simulink model "NREL_5MW_Controller_x86"  (R2019b)
settings: Solver=ode4  StartTime=0.0  StopTime=TMax  FixedStep=DT  MaxStep=DT  RelTol=1e-3  EnableMultiTasking=on
InitFcn:
  | Lambda_ref = 5;
values from neighbouring files (symbols this model uses):
  OutList =     [OutList.mat]
undefined symbols (not defined in the file or in its folder): pitch_cmd, rotor_cmd, strmatch
CloseFcn:
  | olist = OutList;
settings Model: Creator=bjonkman  LastModifiedBy=arthu
settings DataIOCC: SaveFormat=Array  SignalLoggingSaveFormat=ModelDataLogs  SaveOutput=off  SaveTime=off  ReturnWorkspaceOutputs=off  SignalLoggingName=sigsOut
settings OptimizationCC: ExpressionDepthLimit=2147483647  LifeSpan=inf
settings DebuggingCC: SaveWithParameterizedLinksMsg=none  UnderspecifiedInitializationDetection=Classic  MergeDetectMultiDrivingBlocksExec=none  SignalResolutionControl=TryResolveAllWithWarning  MultiTaskDSMMsg=warning  MultiTaskCondExecSysMsg=none  FcnCallInpInsideContextMsg=warning  StateNameClashWarn=warning  SFUnexpectedBacktrackingDiag=warning  SFNoUnconditionalDefaultTransitionDiag=warning  SFExecutionAtInitializationDiag=none  ArithmeticOperatorsInVariantConditions=warning
settings HardwareCC: ProdBitPerPointer=32  ProdBitPerSizeT=32  ProdBitPerPtrDiffT=32  ProdLargestAtomicFloat=None  ProdIntDivRoundTo=Undefined  ProdEndianess=Unspecified  ProdWordSize=32  ProdHWDeviceType=32-bit Generic  TargetUnknown=on
settings ModelReferenceCC: PropagateSignalLabelsOutOfModel=off
settings SFSimCC: SimUseLocalCustomCode=off  CustomCodeUndefinedFunction=UseInterfaceOnly
settings RTWCC: RTWUseLocalCustomCode=off
settings CodeAppCC: StateflowObjectComments=on
settings GRTTargetCC: TargetLangStandard=C89/C90 (ANSI)  ModelReferenceCompliant=off  ParMdlRefBuildCompliant=off  CompOptLevelCompliant=off  ConcurrentExecutionCompliant=off  CombineOutputUpdateFcns=off  MatFileLogging=off  GRTInterface=on
settings ConfigComp: CovMetricSettings=dw  CovHtmlReporting=on  CovSaveCumulativeToWorkspaceVar=on  CovSaveSingleToWorkspaceVar=on  CovExternalEMLEnable=off

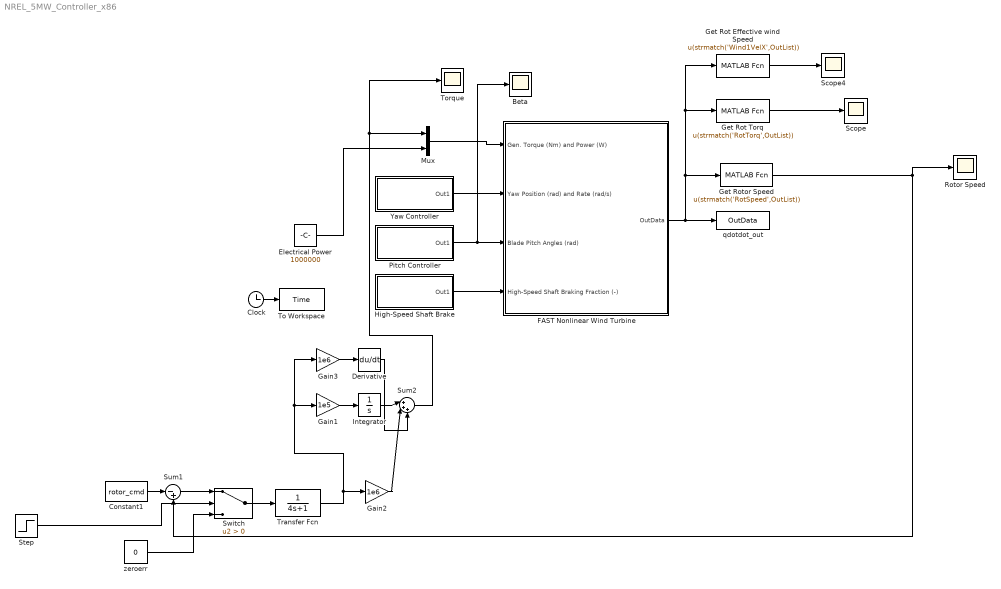
== system NREL_5MW_Controller_x86 ==
  Beta : Scope
  Clock : Clock
  Constant1 : Constant  Value=rotor_cmd
  Derivative : Derivative  CoefficientInTFapproximation=100
  Electrical Power : Constant  Value=1000000
  FAST Nonlinear Wind Turbine : Subsystem  mask(FAST Nonlinear Wind Turbine){}
      mask help: This block contains the FAST S-Function.
      mask init:
      | clear FAST_SFunc
  Gain1 : Gain  Gain=1e5
  Gain2 : Gain  Gain=1e6
  Gain3 : Gain  Gain=1e6
  Get Rot Effective wind Speed : MATLABFcn  MATLABFcn=u(strmatch('Wind1VelX',OutList))
  Get Rot Torq : MATLABFcn  MATLABFcn=u(strmatch('RotTorq',OutList))
  Get Rotor Speed : MATLABFcn  MATLABFcn=u(strmatch('RotSpeed',OutList))
  High-Speed Shaft Brake : Subsystem
  Integrator : Integrator
  Mux : Mux  Inputs=2
  Pitch Controller : Subsystem
  Rotor Speed : Scope
  Scope : Scope
  Scope4 : Scope
  Step : Step  Time=10  Before=-1  SampleTime=0
  Sum1 : Sum  Inputs=|-+
  Sum2 : Sum  Inputs=|+++
  Switch : Switch  Criteria=u2 > Threshold
  To Workspace : ToWorkspace  VariableName=Time  SampleTime=-1
  Torque : Scope
  Transfer Fcn : TransferFcn  Denominator=[4 1]
  Yaw Controller : Subsystem
  qdotdot_out : ToWorkspace  VariableName=OutData  SampleTime=-1
  zeroerr : Constant  Value=0
  wires:
  Clock/1 -> To Workspace/1
  Mux/1 -> FAST Nonlinear Wind Turbine/1(Gen. Torque (Nm) and Power (W))
  Yaw Controller/1(Out1) -> FAST Nonlinear Wind Turbine/2(Yaw Position (rad) and Rate (rad/s))
  Pitch Controller/1(Out1) -> Beta/1, FAST Nonlinear Wind Turbine/3(Blade Pitch Angles (rad))
  High-Speed Shaft Brake/1(Out1) -> FAST Nonlinear Wind Turbine/4(High-Speed Shaft Braking Fraction (-))
  Get Rot Torq/1 -> Scope/1
  FAST Nonlinear Wind Turbine/1(OutData) -> Get Rot Effective wind Speed/1, Get Rot Torq/1, Get Rotor Speed/1, qdotdot_out/1
  Get Rot Effective wind Speed/1 -> Scope4/1
  Electrical Power/1 -> Mux/2
  Constant1/1 -> Sum1/1
  Get Rotor Speed/1 -> Rotor Speed/1, Sum1/2
  Integrator/1 -> Sum2/1
  Gain2/1 -> Sum2/2
  Sum2/1 -> Torque/1, Mux/1
  Gain1/1 -> Integrator/1
  Derivative/1 -> Sum2/3
  Gain3/1 -> Derivative/1
  Sum1/1 -> Switch/1
  Step/1 -> Switch/2
  zeroerr/1 -> Switch/3
  Switch/1 -> Transfer Fcn/1
  Transfer Fcn/1 -> Gain2/1, Gain3/1, Gain1/1

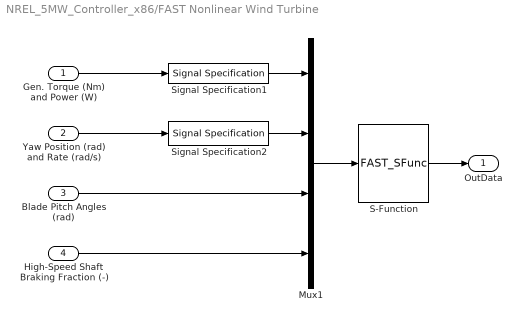
== system NREL_5MW_Controller_x86/FAST Nonlinear Wind Turbine ==
  Gen. Torque (Nm) and Power (W) : Inport
  Yaw Position (rad) and Rate (rad/s) : Inport  Port=2
  Blade Pitch Angles (rad) : Inport  Port=3
  High-Speed Shaft Braking Fraction (-) : Inport  Port=4
  Mux1 : Mux
  S-Function : S-Function  FunctionName=FAST_SFunc  Parameters=FAST_InputFileName, TMax, 0  SFunctionDeploymentMode=off  EnableBusSupport=off
  Signal Specification1 : SignalSpecification  OutDataTypeStr=double  Dimensions=2
  Signal Specification2 : SignalSpecification  OutDataTypeStr=double  Dimensions=2
  OutData : Outport  VectorParamsAs1DForOutWhenUnconnected=off
  wires:
  Gen. Torque (Nm) and Power (W)/1 -> Signal Specification1/1
  S-Function/1 -> OutData/1
  Mux1/1 -> S-Function/1
  Blade Pitch Angles (rad)/1 -> Mux1/3
  Yaw Position (rad) and Rate (rad/s)/1 -> Signal Specification2/1
  Signal Specification1/1 -> Mux1/1
  Signal Specification2/1 -> Mux1/2
  High-Speed Shaft Braking Fraction (-)/1 -> Mux1/4

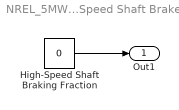
== system NREL_5MW_Controller_x86/High-Speed Shaft Brake ==
  High-Speed Shaft Braking Fraction : Constant  Value=0
  Out1 : Outport  VectorParamsAs1DForOutWhenUnconnected=off
  wires:
  High-Speed Shaft Braking Fraction/1 -> Out1/1

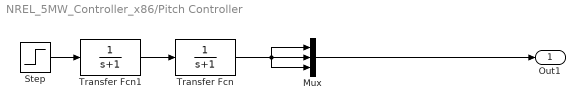
== system NREL_5MW_Controller_x86/Pitch Controller ==
  Mux : Mux  Inputs=3
  Step : Step  Time=0.1  After=pitch_cmd  SampleTime=0
  Transfer Fcn : TransferFcn  Denominator=[1 1]
  Transfer Fcn1 : TransferFcn  Denominator=[1 1]
  Out1 : Outport  VectorParamsAs1DForOutWhenUnconnected=off
  wires:
  Mux/1 -> Out1/1
  Step/1 -> Transfer Fcn1/1
  Transfer Fcn/1 -> Mux/3, Mux/2, Mux/1
  Transfer Fcn1/1 -> Transfer Fcn/1

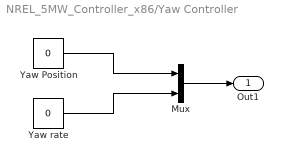
== system NREL_5MW_Controller_x86/Yaw Controller ==
  Mux : Mux  Inputs=2
  Yaw Position : Constant  Value=0
  Yaw rate : Constant  Value=0
  Out1 : Outport  VectorParamsAs1DForOutWhenUnconnected=off
  wires:
  Mux/1 -> Out1/1
  Yaw Position/1 -> Mux/1
  Yaw rate/1 -> Mux/2
